simulink model "filters_for_you"  (R2019b)
settings: Solver=VariableStepAuto  StartTime=0.0  StopTime=10  RelTol=1e-3
undefined symbols (not defined in the file): Discrete, Time
libraries: powerlib_meascontrol x8, dspmlti4 x6, dspxfrm3 x6, dspfdesign x6, visiongeotforms x6, powerlib x4, ctrlSharedLib x3, dspadpt3 x3
settings Model: Creator=Admin  LastModifiedBy=Admin

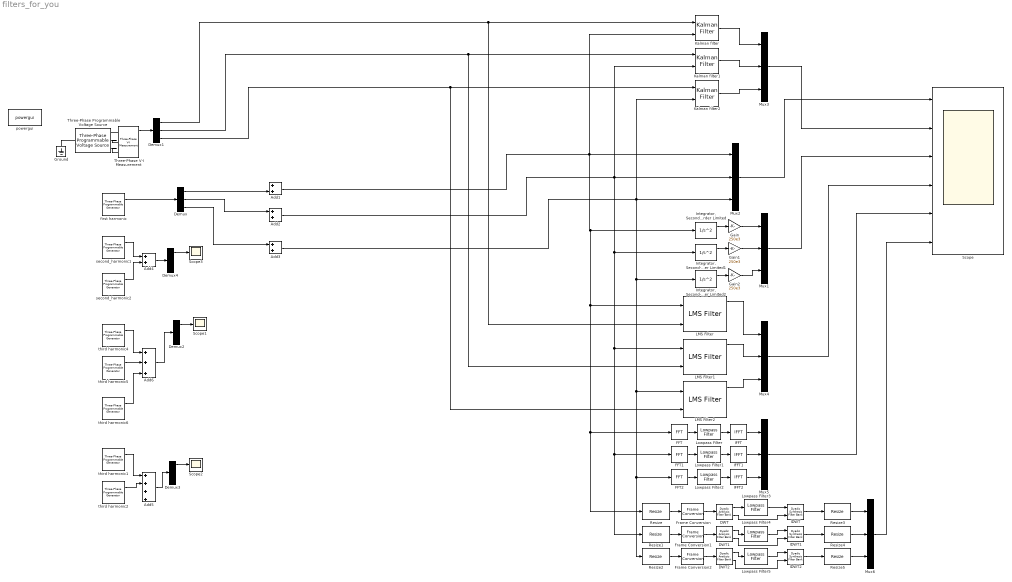
== system filters_for_you ==
  Add{1..4} (4 alike) : Sum
  Add5 : Sum  Inputs=++++
  Add6 : Sum  Inputs=+++
  DWT : dspmlti4/Dyadic Analysis Filter Bank  Wname=Daubechies  OrdRec_ordDec=[1 / 1]  Order=2  LPF="[0.0352   -0.0854   -0.1350   0.4599   0.8069   0.3327]"  HPF="[-0.3327    0.8069   -0.4599   -0.1350    0.0854    0.0352]"  NumLevels=1  tree=Symmetric  Output=Multiple ports  OutputFrames=off
      settings: SourceProductName=DSP System Toolbox  SourceProductBaseCode=DS
  DWT1 : dspmlti4/Dyadic Analysis Filter Bank  Wname=User-defined  OrdRec_ordDec=[1 / 1]  Order=2  LPF="[0.0352   -0.0854   -0.1350   0.4599   0.8069   0.3327]"  HPF="[-0.3327    0.8069   -0.4599   -0.1350    0.0854    0.0352]"  NumLevels=1  tree=Symmetric  Output=Multiple ports  OutputFrames=off
      settings: SourceProductName=DSP System Toolbox  SourceProductBaseCode=DS
  DWT2 : dspmlti4/Dyadic Analysis Filter Bank  Wname=User-defined  OrdRec_ordDec=[1 / 1]  Order=2  LPF="[0.0352   -0.0854   -0.1350   0.4599   0.8069   0.3327]"  HPF="[-0.3327    0.8069   -0.4599   -0.1350    0.0854    0.0352]"  NumLevels=1  tree=Symmetric  Output=Multiple ports  OutputFrames=off
      settings: SourceProductName=DSP System Toolbox  SourceProductBaseCode=DS
  Demux{,1..4} (5 alike) : Demux  Outputs=3
  FFT : dspxfrm3/FFT  FFTImplementation=Auto  CompMethod=Table lookup  TableOpt=NEW  TableOptActive=Speed  BitRevOrder=off  Normalize=off  InheritFFTLength=on  FFTLength=64  WrapInput=on  roundingMode=Floor  overflowMode=off  firstCoeffDataTypeStr=Inherit: Same word length as input  firstCoeffLastDataTypeStr=Inherit: Same word length as input  outputMin=[]  outputMax=[]
  FFT1 : dspxfrm3/FFT  FFTImplementation=Auto  CompMethod=Table lookup  TableOpt=NEW  TableOptActive=Speed  BitRevOrder=off  Normalize=off  InheritFFTLength=on  FFTLength=64  WrapInput=on  roundingMode=Floor  overflowMode=off  firstCoeffDataTypeStr=Inherit: Same word length as input  firstCoeffLastDataTypeStr=Inherit: Same word length as input  outputMin=[]  outputMax=[]
  FFT2 : dspxfrm3/FFT  FFTImplementation=Auto  CompMethod=Table lookup  TableOpt=NEW  TableOptActive=Speed  BitRevOrder=off  Normalize=off  InheritFFTLength=on  FFTLength=64  WrapInput=on  roundingMode=Floor  overflowMode=off  firstCoeffDataTypeStr=Inherit: Same word length as input  firstCoeffLastDataTypeStr=Inherit: Same word length as input  outputMin=[]  outputMax=[]
  Frame Conversion : FrameConversion
  Frame Conversion1 : FrameConversion
  Frame Conversion2 : FrameConversion
  Gain : Gain  Gain=250e3
  Gain1 : Gain  Gain=250e3
  Gain2 : Gain  Gain=250e3
  Ground : powerlib/Elements/Ground  LConnTagsString=a
      settings: SourceProductName=Simscape Electrical
  IDWT : dspmlti4/Dyadic Synthesis Filter Bank  Wname=Daubechies  OrdRec_ordDec=[1 / 1]  Order=2  LPF="[0.3327    0.8069    0.4599   -0.1350   -0.0854    0.0352]"  HPF="[0.0352    0.0854   -0.1350   -0.4599    0.8069   -0.3327]"  NumLevels=1  tree=Symmetric  Input=Multiple ports  OutputFrames=off
      settings: SourceProductName=DSP System Toolbox  SourceProductBaseCode=DS
  IDWT1 : dspmlti4/Dyadic Synthesis Filter Bank  Wname=User-defined  OrdRec_ordDec=[1 / 1]  Order=2  LPF="[0.3327    0.8069    0.4599   -0.1350   -0.0854    0.0352]"  HPF="[0.0352    0.0854   -0.1350   -0.4599    0.8069   -0.3327]"  NumLevels=1  tree=Symmetric  Input=Multiple ports  OutputFrames=off
      settings: SourceProductName=DSP System Toolbox  SourceProductBaseCode=DS
  IDWT2 : dspmlti4/Dyadic Synthesis Filter Bank  Wname=User-defined  OrdRec_ordDec=[1 / 1]  Order=2  LPF="[0.3327    0.8069    0.4599   -0.1350   -0.0854    0.0352]"  HPF="[0.0352    0.0854   -0.1350   -0.4599    0.8069   -0.3327]"  NumLevels=1  tree=Symmetric  Input=Multiple ports  OutputFrames=off
      settings: SourceProductName=DSP System Toolbox  SourceProductBaseCode=DS
  IFFT : dspxfrm3/IFFT  FFTImplementation=Auto  CompMethod=Table lookup  TableOpt=NEW  TableOptActive=Speed  BitRevOrder=off  cs_in=off  Normalize=on  InheritFFTLength=on  FFTLength=64  WrapInput=on  mode=Complex  outSamplingMode=Sample based  roundingMode=Floor  overflowMode=off  firstCoeffDataTypeStr=Inherit: Same word length as input  firstCoeffLastDataTypeStr=Inherit: Same word length as input  outputMin=[]  outputMax=[]
      settings: SourceProductName=DSP System Toolbox
  IFFT1 : dspxfrm3/IFFT  FFTImplementation=Auto  CompMethod=Table lookup  TableOpt=NEW  TableOptActive=Speed  BitRevOrder=off  cs_in=off  Normalize=on  InheritFFTLength=on  FFTLength=64  WrapInput=on  mode=Complex  outSamplingMode=Sample based  roundingMode=Floor  overflowMode=off  firstCoeffDataTypeStr=Inherit: Same word length as input  firstCoeffLastDataTypeStr=Inherit: Same word length as input  outputMin=[]  outputMax=[]
      settings: SourceProductName=DSP System Toolbox
  IFFT2 : dspxfrm3/IFFT  FFTImplementation=Auto  CompMethod=Table lookup  TableOpt=NEW  TableOptActive=Speed  BitRevOrder=off  cs_in=off  Normalize=on  InheritFFTLength=on  FFTLength=64  WrapInput=on  mode=Complex  outSamplingMode=Sample based  roundingMode=Floor  overflowMode=off  firstCoeffDataTypeStr=Inherit: Same word length as input  firstCoeffLastDataTypeStr=Inherit: Same word length as input  outputMin=[]  outputMax=[]
      settings: SourceProductName=DSP System Toolbox
  "Integrator, Second-Order Limited" : SecondOrderIntegrator  LimitX=on  UpperLimitX=1  LowerLimitX=0  LimitDXDT=on
  "Integrator, Second-Order Limited1" : SecondOrderIntegrator  LimitX=on  UpperLimitX=1  LowerLimitX=0  LimitDXDT=on
  "Integrator, Second-Order Limited2" : SecondOrderIntegrator  LimitX=on  UpperLimitX=1  LowerLimitX=0  LimitDXDT=on
  Kalman filter : ctrlSharedLib/Kalman Filter  TimeDomain=Discrete-Time  UseCurrentEstimator=on  ModelSource=LTI State-Space Variable  ModelSourceVariable=ss(0.95,1,1,0, 0.0001)  A=0.95  B=1  C=1  D=0  NumberOfStates=1  NumberOfInputs=1  NumberOfOutputs=1  InitialEstimateSource=Dialog  X0=0  P0=10  UseK=off  UseGH=on  NumberOfProcessNoiseInputs=1  G=1  TimeInvariantG=on  H=0  TimeInvariantH=on  Q=0.05  TimeInvariantQ=on  R=1  TimeInvariantR=on  N=0  TimeInvariantN=on  AddInputPort=on  AddEnablePort=off  OutputEstimatedY=off  OutputP=off  Ts=-1
      settings: SourceProductBaseCode=CT
  Kalman filter1 : ctrlSharedLib/Kalman Filter  TimeDomain=Discrete-Time  UseCurrentEstimator=on  ModelSource=LTI State-Space Variable  ModelSourceVariable=ss(0.95,1,1,0,0.0001)  A=0.95  B=1  C=1  D=0  NumberOfStates=1  NumberOfInputs=1  NumberOfOutputs=1  InitialEstimateSource=Dialog  X0=0  P0=10  UseK=off  UseGH=on  NumberOfProcessNoiseInputs=1  G=1  TimeInvariantG=on  H=0  TimeInvariantH=on  Q=0.05  TimeInvariantQ=on  R=1  TimeInvariantR=on  N=0  TimeInvariantN=on  AddInputPort=on  AddEnablePort=off  OutputEstimatedY=off  OutputP=off  Ts=-1
      settings: SourceProductBaseCode=CT
  Kalman filter2 : ctrlSharedLib/Kalman Filter  TimeDomain=Discrete-Time  UseCurrentEstimator=on  ModelSource=LTI State-Space Variable  ModelSourceVariable=ss(0.95,1,1,0,0.0001)  A=0.95  B=1  C=1  D=0  NumberOfStates=1  NumberOfInputs=1  NumberOfOutputs=1  InitialEstimateSource=Dialog  X0=0  P0=10  UseK=off  UseGH=on  NumberOfProcessNoiseInputs=1  G=1  TimeInvariantG=on  H=0  TimeInvariantH=on  Q=0.05  TimeInvariantQ=on  R=1  TimeInvariantR=on  N=0  TimeInvariantN=on  AddInputPort=on  AddEnablePort=off  OutputEstimatedY=off  OutputP=off  Ts=-1
      settings: SourceProductBaseCode=CT
  LMS Filter : dspadpt3/LMS Filter  Algo=Normalized LMS  L=32  stepflag=Dialog  mu=0.1  leakage=1.0  ic=0  Adapt=off  resetflag=None  weights=on  addnparflag=off  roundingMode=Floor  overflowMode=off
      settings: SourceProductName=DSP System Toolbox  SourceProductBaseCode=DS
  LMS Filter1 : dspadpt3/LMS Filter  Algo=Normalized LMS  L=32  stepflag=Dialog  mu=0.1  leakage=1.0  ic=0  Adapt=off  resetflag=None  weights=on  addnparflag=off  roundingMode=Floor  overflowMode=off
      settings: SourceProductName=DSP System Toolbox  SourceProductBaseCode=DS
  LMS Filter2 : dspadpt3/LMS Filter  Algo=Normalized LMS  L=32  stepflag=Dialog  mu=0.1  leakage=1.0  ic=0  Adapt=off  resetflag=None  weights=on  addnparflag=off  roundingMode=Floor  overflowMode=off
      settings: SourceProductName=DSP System Toolbox  SourceProductBaseCode=DS
  Lowpass Filter{,1..5} (6 alike) : dspfdesign/Lowpass Filter  FilterType=FIR  DesignForMinimumOrder=on  FilterOrder=50  PassbandFrequency=60  StopbandFrequency=1000  PassbandRipple=0.1  StopbandAttenuation=80  InheritSampleRate=off  SampleRate=44100  SimulateUsing=Interpreted execution  roundingMode=Floor  coeffsDataTypeStr=fixdt(1,16)
  Mux{1..6} (6 alike) : Mux  Inputs=3
  Resize : visiongeotforms/Resize  specify=Output size as a percentage of input size  rfactor=[200 150]  outCols=25  outRows=25  outRowsCols=[25 35]  interp_method=Bilinear  antialias=on  useROI=off  roiFlag=off  roundingMode=Nearest  overflowMode=on  prodOutputMode=Binary point scaling  prodOutputWordLength=32  prodOutputFracLength=10  prodOutputSlope=2^-10  accumSlope=2^-10  outputSlope=2^-10
      settings: SourceProductName=Computer Vision Toolbox  SourceProductBaseCode=VP
  Resize1 : visiongeotforms/Resize  specify=Output size as a percentage of input size  rfactor=[200 150]  outCols=25  outRows=25  outRowsCols=[25 35]  interp_method=Bilinear  antialias=on  useROI=off  roiFlag=off  roundingMode=Nearest  overflowMode=on  prodOutputMode=Binary point scaling  prodOutputWordLength=32  prodOutputFracLength=10  prodOutputSlope=2^-10  accumSlope=2^-10  outputSlope=2^-10
      settings: SourceProductName=Computer Vision Toolbox  SourceProductBaseCode=VP
  Resize2 : visiongeotforms/Resize  specify=Output size as a percentage of input size  rfactor=[200 150]  outCols=25  outRows=25  outRowsCols=[25 35]  interp_method=Bilinear  antialias=on  useROI=off  roiFlag=off  roundingMode=Nearest  overflowMode=on  prodOutputMode=Binary point scaling  prodOutputWordLength=32  prodOutputFracLength=10  prodOutputSlope=2^-10  accumSlope=2^-10  outputSlope=2^-10
      settings: SourceProductName=Computer Vision Toolbox  SourceProductBaseCode=VP
  Resize3 : visiongeotforms/Resize  specify=Number of output rows and preserve aspect ratio  rfactor=[200 150]  outCols=25  outRows=1  outRowsCols=[25 35]  interp_method=Bilinear  antialias=on  useROI=off  roiFlag=off  roundingMode=Nearest  overflowMode=on  prodOutputMode=Binary point scaling  prodOutputWordLength=32  prodOutputFracLength=10  prodOutputSlope=2^-10  accumSlope=2^-10  outputSlope=2^-10
      settings: SourceProductName=Computer Vision Toolbox  SourceProductBaseCode=VP
  Resize4 : visiongeotforms/Resize  specify=Number of output rows and preserve aspect ratio  rfactor=[200 150]  outCols=25  outRows=1  outRowsCols=[25 35]  interp_method=Bilinear  antialias=on  useROI=off  roiFlag=off  roundingMode=Nearest  overflowMode=on  prodOutputMode=Binary point scaling  prodOutputWordLength=32  prodOutputFracLength=10  prodOutputSlope=2^-10  accumSlope=2^-10  outputSlope=2^-10
      settings: SourceProductName=Computer Vision Toolbox  SourceProductBaseCode=VP
  Resize5 : visiongeotforms/Resize  specify=Number of output rows and preserve aspect ratio  rfactor=[200 150]  outCols=25  outRows=1  outRowsCols=[25 35]  interp_method=Bilinear  antialias=on  useROI=off  roiFlag=off  roundingMode=Nearest  overflowMode=on  prodOutputMode=Binary point scaling  prodOutputWordLength=32  prodOutputFracLength=10  prodOutputSlope=2^-10  accumSlope=2^-10  outputSlope=2^-10
      settings: SourceProductName=Computer Vision Toolbox  SourceProductBaseCode=VP
  Scope : Scope  NumInputPorts=6
  Scope1 : Scope
  Scope2 : Scope
  Scope3 : Scope
  Three-Phase Programmable Voltage Source : powerlib/Electrical Sources/Three-Phase Programmable Voltage Source  PositiveSequence="[250e3  0 60]"  VariationEntity=None  VariationType=Table of time-amplitude pairs  VariationTypeAlt=Step  VariationStep=0.5  VariationRate=10  VariationMagnitude=0.3  VariationFrequency=2  VariationTiming=[1 2]  VariationPhaseA=off  Amplitudes=[1 0.8 1.2 1.0]  TimeValues=[0 0.1 0.15 0.2]  HarmonicGeneration=off  HarmonicA=[3 0.2 -25 0]  HarmonicB=[2 0.15 35 2]  Timing="[0.05  3]"  BusType=swing  Pref=0  Qref=0  Qmin=-inf  Qmax=inf
      settings: SourceProductName=Simscape Electrical
  Three-Phase V-I Measurement : powerlib/Measurements/Three-Phase V-I Measurement  VoltageMeasurement=phase-to-ground  SetLabelV=off  LabelV=Vabc  Vpu=off  VpuLL=off  CurrentMeasurement=yes  SetLabelI=off  LabelI=Iabc  Ipu=off  Pbase=100e6  Vbase=500e3  OutputType=Complex  PhasorSimulation=off  PSBequivalent=0
      settings: SourceProductName=Simscape Electrical
  first harmonic : powerlib_meascontrol/Pulse & Signal Generators/Three-Phase Programmable Generator  Par_Vps=[250e3, 0, 60]  VariationEntity=None  VariationType=Ramp  VariationStep=-0.5  VariationRate=10  VariationMag=0.3  VariationFreq=2  Par_Timing_Variation="[0.2  1.2]"  SinglePhase=on  Yampli=[1 0.2 1.2 1.0]  Xtime=[0 0.1 0.15 0.2]  HarmonicGeneration=on  Par_HarmoA="[3  90e3  -25 0]"  Par_HarmoB="[3  90e3  35  2]"  Par_Timing_Harmo="[ 0.05  99]"  Ts=0.0001
      settings: SourceProductName=Simscape Electrical  SourceProductBaseCode=PS
  powergui : powerlib/powergui  Priority=1  SimulationMode=Discrete  SampleTime=0.0001  frequency=60  Iterations=50  frequencyindice=60  Pbase=100e6  ErrMax=1e-4  UnitsV=kV  UnitsW=MW  buscounter=0  FunctionMessages=off  echomessages=off  EnableUseOfTLC=off  CurrentSourceSwitches=off  DisableSnubberDevices=off  DisableRonSwitches=off  DisableVfSwitches=off  DisplayEquations=off  AutomaticDiscreteSolvers=off  SolverType=Tustin/Backward Euler (TBE)  Interpol=off  ExternalGateDelay=off  methode=off  Ts=100  x0status=blocks  SPID=on  SwTol=0  HookPort=off  NonlinearTolerance=1e-4  nMaxIteration=100  ContinueOnMaxIteration=off  RestoreLinks=warning  ResistiveCurrentMeasurement=off  Frange=[0:2:500]  Ylog=off  Xlog=on  ShowGrid=off  save=off  variable=ZData  structure=0  ZoomFFT=off  StartTime=0.0  cycles=1  DisplayStyle=1  fundamental=60  FreqAxis=off  MaxFrequency=1000  frequencyindicesteady=1  RmsSteady=1  display=off
      settings: SourceProductName=Simscape Electrical
  second_harmonic1 : powerlib_meascontrol/Pulse & Signal Generators/Three-Phase Programmable Generator  Par_Vps=[250e3, 0, 60]  VariationEntity=None  VariationType=Ramp  VariationStep=-0.5  VariationRate=10  VariationMag=0.3  VariationFreq=2  Par_Timing_Variation="[0.2  1.2]"  SinglePhase=on  Yampli=[1 0.2 1.2 1.0]  Xtime=[0 0.1 0.15 0.2]  HarmonicGeneration=on  Par_HarmoA="[15  90e2  -25 1]"  Par_HarmoB="[15  90e2  35  1]"  Par_Timing_Harmo="[ 0.05  99]"  Ts=0.0001
      settings: SourceProductName=Simscape Electrical  SourceProductBaseCode=PS
  second_harmonic2 : powerlib_meascontrol/Pulse & Signal Generators/Three-Phase Programmable Generator  Par_Vps=[250e3, 0, 60]  VariationEntity=None  VariationType=Ramp  VariationStep=-0.5  VariationRate=10  VariationMag=0.3  VariationFreq=2  Par_Timing_Variation="[0.2  1.2]"  SinglePhase=on  Yampli=[1 0.2 1.2 1.0]  Xtime=[0 0.1 0.15 0.2]  HarmonicGeneration=on  Par_HarmoA="[50  100e2  -25 1]"  Par_HarmoB="[50  100e3  35  1]"  Par_Timing_Harmo="[ 0.05  99]"  Ts=0.0001
      settings: SourceProductName=Simscape Electrical  SourceProductBaseCode=PS
  third harmonic1 : powerlib_meascontrol/Pulse & Signal Generators/Three-Phase Programmable Generator  Par_Vps=[250e3, 0, 60]  VariationEntity=None  VariationType=Ramp  VariationStep=-0.5  VariationRate=10  VariationMag=0.3  VariationFreq=2  Par_Timing_Variation="[0.2  1.2]"  SinglePhase=on  Yampli=[1 0.2 1.2 1.0]  Xtime=[0 0.1 0.15 0.2]  HarmonicGeneration=on  Par_HarmoA="[15  90e3  -25 1]"  Par_HarmoB="[15  90e3  35  1]"  Par_Timing_Harmo="[ 0.05  99]"  Ts=0.0001
      settings: SourceProductName=Simscape Electrical  SourceProductBaseCode=PS
  third harmonic2 : powerlib_meascontrol/Pulse & Signal Generators/Three-Phase Programmable Generator  Par_Vps=[250e3, 0, 60]  VariationEntity=None  VariationType=Ramp  VariationStep=-0.5  VariationRate=10  VariationMag=0.3  VariationFreq=2  Par_Timing_Variation="[0.2  1.2]"  SinglePhase=on  Yampli=[1 0.2 1.2 1.0]  Xtime=[0 0.1 0.15 0.2]  HarmonicGeneration=on  Par_HarmoA="[100  100e2  -25 1]"  Par_HarmoB="[100  100e3  35  1]"  Par_Timing_Harmo="[ 0.05  99]"  Ts=0.0001
      settings: SourceProductName=Simscape Electrical  SourceProductBaseCode=PS
  third harmonic4 : powerlib_meascontrol/Pulse & Signal Generators/Three-Phase Programmable Generator  Par_Vps=[250e3, 0, 60]  VariationEntity=None  VariationType=Ramp  VariationStep=-0.5  VariationRate=10  VariationMag=0.3  VariationFreq=2  Par_Timing_Variation="[0.2  1.2]"  SinglePhase=on  Yampli=[1 0.2 1.2 1.0]  Xtime=[0 0.1 0.15 0.2]  HarmonicGeneration=on  Par_HarmoA="[15  90e2  -25 1]"  Par_HarmoB="[15  90e2  35  1]"  Par_Timing_Harmo="[ 0.05  99]"  Ts=0.0001
      settings: SourceProductName=Simscape Electrical  SourceProductBaseCode=PS
  third harmonic5 : powerlib_meascontrol/Pulse & Signal Generators/Three-Phase Programmable Generator  Par_Vps=[250e3, 0, 60]  VariationEntity=None  VariationType=Ramp  VariationStep=-0.5  VariationRate=10  VariationMag=0.3  VariationFreq=2  Par_Timing_Variation="[0.2  1.2]"  SinglePhase=on  Yampli=[1 0.2 1.2 1.0]  Xtime=[0 0.1 0.15 0.2]  HarmonicGeneration=on  Par_HarmoA="[50  100e2  -25 1]"  Par_HarmoB="[50  100e3  35  1]"  Par_Timing_Harmo="[ 0.05  99]"  Ts=0.0001
      settings: SourceProductName=Simscape Electrical  SourceProductBaseCode=PS
  third harmonic6 : powerlib_meascontrol/Pulse & Signal Generators/Three-Phase Programmable Generator  Par_Vps=[250e3, 0, 60]  VariationEntity=None  VariationType=Ramp  VariationStep=-0.5  VariationRate=10  VariationMag=0.3  VariationFreq=2  Par_Timing_Variation="[0.2  1.2]"  SinglePhase=on  Yampli=[1 0.2 1.2 1.0]  Xtime=[0 0.1 0.15 0.2]  HarmonicGeneration=on  Par_HarmoA="[3  100e2  -25 1]"  Par_HarmoB="[3  100e3  35  1]"  Par_Timing_Harmo="[ 0.05  99]"  Ts=0.0001
      settings: SourceProductName=Simscape Electrical  SourceProductBaseCode=PS
  wires:
  Kalman filter1/1 -> Mux3/2
  Kalman filter/1 -> Mux3/1
  Kalman filter2/1 -> Mux3/3
  "Integrator, Second-Order Limited"/1 -> Gain/1
  LMS Filter/1 -> Mux4/1
  LMS Filter1/1 -> Mux4/2
  LMS Filter2/1 -> Mux4/3
  Gain/1 -> Mux1/1
  "Integrator, Second-Order Limited1"/1 -> Gain1/1
  Gain1/1 -> Mux1/2
  "Integrator, Second-Order Limited2"/1 -> Gain2/1
  Gain2/1 -> Mux1/3
  Mux2/1 -> Scope/1
  Mux3/1 -> Scope/2
  Mux1/1 -> Scope/3
  Mux4/1 -> Scope/4
  Mux5/1 -> Scope/5
  FFT/1 -> Lowpass Filter/1
  FFT1/1 -> Lowpass Filter1/1
  FFT2/1 -> Lowpass Filter2/1
  Mux6/1 -> Scope/6
  Lowpass Filter/1 -> IFFT/1
  IFFT/1 -> Mux5/1
  Lowpass Filter1/1 -> IFFT1/1
  Lowpass Filter2/1 -> IFFT2/1
  IFFT1/1 -> Mux5/2
  IFFT2/1 -> Mux5/3
  Resize/1 -> Frame Conversion/1
  Frame Conversion/1 -> DWT/1
  DWT/1 -> Lowpass Filter3/1
  Resize1/1 -> Frame Conversion1/1
  Resize2/1 -> Frame Conversion2/1
  Frame Conversion1/1 -> DWT1/1
  Frame Conversion2/1 -> DWT2/1
  DWT1/1 -> Lowpass Filter4/1
  DWT2/1 -> Lowpass Filter5/1
  Lowpass Filter3/1 -> IDWT/1
  IDWT/1 -> Resize3/1
  DWT/2 -> IDWT/2
  IDWT2/1 -> Resize5/1
  Resize5/1 -> Mux6/3
  Resize4/1 -> Mux6/2
  IDWT1/1 -> Resize4/1
  Lowpass Filter4/1 -> IDWT1/1
  Lowpass Filter5/1 -> IDWT2/1
  DWT1/2 -> IDWT1/2
  DWT2/2 -> IDWT2/2
  Resize3/1 -> Mux6/1
  Demux/1 -> Add1/2
  Demux/2 -> Add2/1
  Demux/3 -> Add3/1
  Add1/1 -> Resize/1, FFT/1, LMS Filter/1, "Integrator, Second-Order Limited"/1, Kalman filter/2, Mux2/1
  Add2/1 -> Resize1/1, FFT1/1, LMS Filter1/1, "Integrator, Second-Order Limited1"/1, Kalman filter1/2, Mux2/2
  Add3/1 -> Resize2/1, FFT2/1, LMS Filter2/1, "Integrator, Second-Order Limited2"/1, Kalman filter2/2, Mux2/3
  first harmonic/1 -> Demux/1
  Three-Phase V-I Measurement/1 -> Demux1/1
  Demux1/1 -> LMS Filter/2, Kalman filter/1
  Demux1/2 -> LMS Filter1/2, Kalman filter1/1
  Demux1/3 -> LMS Filter2/2, Kalman filter2/1
  second_harmonic1/1 -> Add4/1
  second_harmonic2/1 -> Add4/2
  third harmonic2/1 -> Add5/2
  Demux3/1 -> Scope2/1
  Add5/1 -> Demux3/1
  third harmonic1/1 -> Add5/1
  third harmonic4/1 -> Add6/1
  third harmonic5/1 -> Add6/2
  third harmonic6/1 -> Add6/3
  Demux2/1 -> Scope1/1
  Add6/1 -> Demux2/1
  Add4/1 -> Demux4/1
  Demux4/1 -> Scope3/1
  connections:
  Ground/LConn1 -- Three-Phase Programmable Voltage Source/LConn1
  Three-Phase V-I Measurement/LConn1 -- Three-Phase Programmable Voltage Source/RConn1
  Three-Phase Programmable Voltage Source/RConn2 -- Three-Phase V-I Measurement/LConn2
  Three-Phase Programmable Voltage Source/RConn3 -- Three-Phase V-I Measurement/LConn3
